simulink model "sgMdl_IO145_AnalogDigitalLoopback"  (R2024b)
settings: Solver=FixedStepAuto  StartTime=0.0  StopTime=inf  RelTol=1e-3  EnableMultiTasking=on
libraries: speedgoatlib_IO145 x5
Description:
  | IO145 - Analog and Digital Loopback
settings Model: ModifiedByFormat=Speedgoat  SimulationMode=external  ExtModeEnableFloating=off  ExtModeTrigDuration=100000  Creator=Speedgoat  LastModifiedBy=Speedgoat
settings SolverCC: ConcurrentTasks=on  AlgebraicLoopSolver=TrustRegion  PositivePriorityOrder=on
settings DataIOCC: SaveFormat=StructureWithTime  ReturnWorkspaceOutputs=off
settings OptimizationCC: BlockReduction=off  OptimizeBlockIOStorage=off  BufferReuse=off  ReuseModelBlockBuffer=off  GlobalBufferReuse=off  ExpressionFolding=off  LocalBlockOutputs=off
settings DebuggingCC: TasksWithSamePriorityMsg=none  UnconnectedInputMsg=warning  UnconnectedOutputMsg=warning  UnconnectedLineMsg=warning  SFExecutionAtInitializationDiag=none  ArithmeticOperatorsInVariantConditions=warning
settings HardwareCC: ProdBitPerLong=64  ProdLongLongMode=on  ProdHWDeviceType=Intel->x86-64 (Linux 64)
settings ModelReferenceCC: EnableRefExpFcnMdlSchedulingChecks=on
settings SFSimCC: SimUseLocalCustomCode=off  CustomCodeUndefinedFunction=UseInterfaceOnly
settings RTWCC: Description=Speedgoat Real-Time Target Machine  SystemTargetFile=speedgoat.tlc  TemplateMakefile=slrealtime_default_tmf  RTWUseLocalCustomCode=off  Toolchain=Simulink Real-Time Toolchain  BuildConfiguration=Faster Runs  TargetLang=C++  GPUComputeCapability=3.5  DLArmComputeVersion=19.05
settings CodeAppCC: StateflowObjectComments=on
settings SimulinkRealTimeTargetCC: SubcomponentCodeInterfacePackaging=Reusable function  InstructionSetFMA=off  LogToMDFFile=off  SLRTFileLogMaxRuns=10  UseGCCFastMath=on
settings ConfigComp: CovBoundaryAbsTol=1.0e-5
settings SimscapeCC: SimscapeNormalizeSystem=off

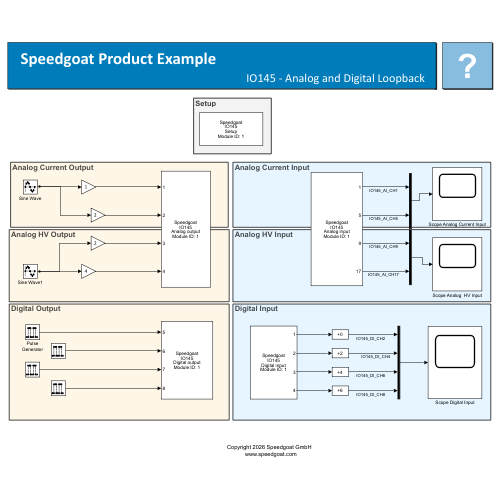
[thumbnail: Simulink's stored preview of the top-level diagram]
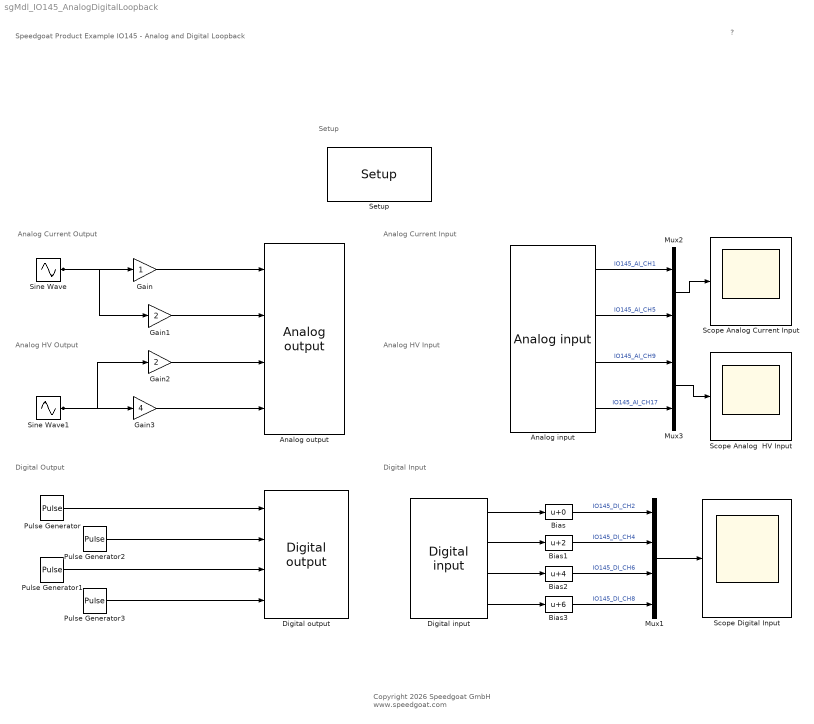
== system sgMdl_IO145_AnalogDigitalLoopback ==
  note: Digital Input
  note: Analog HV Input
  note: Analog HV Output
  note: Digital Output
  note: Setup
  note: Analog Current Output
  note: Analog Current Input
  note: Speedgoat Product Example
      | IO145 - Analog and Digital Loopback
  note: ?
  note: Copyright 2026 Speedgoat GmbH
      |  www.speedgoat.com
  "Analog input " : speedgoatlib_IO145/Analog input   parModuleId=1  parSampleTime=-1  parPciSlot=-1  parAdcChannels=[1 9 17 25]  parAdcNumActiveChannels=[1 1 1 1]  parAdcVoltageRange=[1 1 1 1 1 1 1 1 1 1 1 1 1 1 1 1 1 1 1 1 1 1 1 1 1 1 1 1 1 1 1 1]  parAdcCoupling=[1 1 1 1]  parAdcContSampling=0  parAdcDmaEnable=0  parAdcActiveDmaDevices=[1 1 1 1]  parAdcFrameSize=100
      settings: SourceProductName=Simulink Real-Time: Speedgoat I/O Blockset
  "Analog output " : speedgoatlib_IO145/Analog output   parModuleId=1  parSampleTime=-1  parPciSlot=-1  parDacChannels=[1 2 3 4]  parDacVoltageRange=[10 10 7 7 7 7 1 1]  parDacOverRange=[0 0 0 0 0 0 0 0]  parDacInitValues=[0 0 0 0]  parDacReset=[1 1 1 1]  parDacSyncOut=1  parDacDmaEnable=0  parDacActiveDmaDevices=[1 1 1 1]  parDacDmaLatency=2  parDacFrameSize=100
      settings: SourceProductName=Simulink Real-Time: Speedgoat I/O Blockset
  Bias : Bias  SaturateOnIntegerOverflow=off
  Bias1 : Bias  Bias=2  SaturateOnIntegerOverflow=off
  Bias2 : Bias  Bias=4  SaturateOnIntegerOverflow=off
  Bias3 : Bias  Bias=6  SaturateOnIntegerOverflow=off
  "Digital input " : speedgoatlib_IO145/Digital input   parModuleId=1  parSampleTime=-1  parPciSlot=-1  parDiChannels=[2 4 6 8]
      settings: SourceProductName=Simulink Real-Time: Speedgoat I/O Blockset
  "Digital output " : speedgoatlib_IO145/Digital output   parModuleId=1  parSampleTime=-1  parPciSlot=-1  parDoChannels=[1 3 5 7]  parDoInitValues=[0 0 0 0]  parDoReset=[1 1 1 1]
      settings: SourceProductName=Simulink Real-Time: Speedgoat I/O Blockset
  Gain : Gain
  Gain1 : Gain  Gain=2
  Gain2 : Gain  Gain=2
  Gain3 : Gain  Gain=4
  Mux1 : Mux
  Mux2 : Mux  Inputs=2
  Mux3 : Mux  Inputs=2
  Pulse Generator : DiscretePulseGenerator  Period=25  PulseWidth=5  SampleTime=0.001
  Pulse Generator1 : DiscretePulseGenerator  Period=25  PulseWidth=15  SampleTime=0.001
  Pulse Generator2 : DiscretePulseGenerator  Period=25  PulseWidth=10  SampleTime=0.001
  Pulse Generator3 : DiscretePulseGenerator  Period=25  PulseWidth=20  SampleTime=0.001
  Scope Analog  HV Input : Scope
  Scope Analog Current Input : Scope
  Scope Digital Input : Scope
  "Setup " : speedgoatlib_IO145/Setup   parPciSlot=-1  parModuleId=1  parInterModuleSync=Independent  parConvClockBaseRate=20MHz  parConvClock1Divider=20000  parConvClock2Divider=20000  parFrameTriggerEnable=off  parFrameTriggerDivider=10  parConvClock1BaseRate=1  parConvClock2BaseRate=1  parFrameTriggerClock=1  parAdcCoupling1=Differential  parAdcChannels1=[1 2]  parAdcChannel11=on  parAdcChannel12=off  parAdcChannel13=off  parAdcChannel14=off  parAdcChannel15=off  parAdcChannel16=off  parAdcChannel17=off  parAdcChannel18=off  parAdcRangeAll1=+-25 mA  parVoltageRangePerChannelEn1=off  parAdcRange11=+-25 mA  parAdcRange12=+-25 mA  parAdcRange13=+-25 mA  parAdcRange14=+-25 mA  parAdcRange15=+-25 mA  parAdcRange16=+-25 mA  parAdcRange17=+-25 mA  parAdcRange18=+-25 mA  parAdcCoupling2=Differential  parAdcChannels2=[9 10]  parAdcChannel21=on  parAdcChannel22=off  parAdcChannel23=off  parAdcChannel24=off  parAdcChannel25=off  parAdcChannel26=off  parAdcChannel27=off  parAdcChannel28=off  parAdcRangeAll2=+-25 mA  parVoltageRangePerChannelEn2=off  parAdcRange21=+-25 mA  parAdcRange22=+-25 mA  parAdcRange23=+-25 mA  parAdcRange24=+-25 mA  parAdcRange25=+-25 mA  parAdcRange26=+-25 mA  parAdcRange27=+-25 mA  parAdcRange28=+-25 mA  parAdcCoupling3=Differential  parAdcChannels3=[17 18]  parAdcChannel31=on  parAdcChannel32=off  parAdcChannel33=off  parAdcChannel34=off  parAdcChannel35=off  parAdcChannel36=off  parAdcChannel37=off  parAdcChannel38=off  parAdcRangeAll3=+-10V  parVoltageRangePerChannelEn3=off  parAdcRange31=+-20V  parAdcRange32=+-10V  parAdcRange33=+-10V  parAdcRange34=+-10V  parAdcRange35=+-10V  parAdcRange36=+-10V  parAdcRange37=+-10V  parAdcRange38=+-10V  parAdcCoupling4=Differential  parAdcChannels4=[25 26]  parAdcChannel41=on  parAdcChannel42=off  parAdcChannel43=off  parAdcChannel44=off  parAdcChannel45=off  parAdcChannel46=off  parAdcChannel47=off  parAdcChannel48=off  parAdcRangeAll4=+-10V  parVoltageRangePerChannelEn4=off  parAdcRange41=+-10V  parAdcRange42=+-10V  parAdcRange43=+-10V  parAdcRange44=+-10V  parAdcRange45=+-10V  parAdcRange46=+-10V  parAdcRange47=+-10V  parAdcRange48=+-10V  parAdcChannels=[1 9 17 25]  parAdcNumActiveChannels=[1 1 1 1]  parAdcVoltageRange=[1 1 1 1 1 1 1 1 1 1 1 1 1 1 1 1 1 1 1 1 1 1 1 1 1 1 1 1 1 1 1 1]  parAdcCoupling=[1 1 1 1]  parAdcContSampling=off  parAdcAutoCorrection=on  parAdcDmaEnable=off  parAdcDmaClock=Clock 1  parAdcFrameSize_=100  parAdcSampleTime_=-1  parAdcActiveDmaDevices=[1 1 1 1]  parAdcFrameTriggerEnable=0  parAdcFrameSize=100  parAdcSampleTime=0.1  parDacChannels=[1 2 3 4]  parDacChannel1=on  parDacChannel2=on  parDacChannel3=on  parDacChannel4=on  parDacChannel5=off  parDacChannel6=off  parDacChannel7=off  parDacChannel8=off  parDacInitValues=0  parDacResets=1  parDacVoltageRange=[10 10 7 7 7 7 1 1]  parDacOverRange=[0 0 0 0 0 0 0 0]  parDacRange1=0-20 mA  parDacInitValue1=0  parDacReset1=on  parDacRange2=0-20 mA  parDacInitValue2=0  parDacReset2=on  parDacRange3=+-10 V  parDacInitValue3=0  parDacReset3=on  parDacRange4=+-10 V  parDacInitValue4=0  parDacReset4=on  parDacRange5=+-10 V  parDacInitValue5=0  parDacReset5=on  parDacRange6=+-10 V  parDacInitValue6=0  parDacReset6=on  parDacRange7=0-5 V  parDacInitValue7=0  parDacReset7=on  parDacRange8=0-5 V  parDacInitValue8=0  parDacReset8=on  parDacAutoCorrection=on  parDacSyncOut=on  parDacDmaEnable=off  parDacDmaLatency=Until next frame  parDacDmaClock=Clock 1  parDacFrameSize_=100  parDacSampleTime_=-1  parDacActiveDmaDevices=[1 1 1 1]  parDacFrameTriggerEnable=0  parDacFrameSize=100  parDacSampleTime=0.1  parDiChannels=[2 4 6 8]  parDoChannels=[1 3 5 7]  parDioChannel1=Out  parDioChannel2=In  parDioChannel3=Out  parDioChannel4=In  parDioChannel5=Out  parDioChannel6=In  parDioChannel7=Out  parDioChannel8=In  parDoInitValues=[0 0 0 0]  parDoReset=[1 1 1 1]  parDoInitValue1=0  parDoReset1=on  parDoInitValue2=0  parDoReset2=on  parDoInitValue3=0  parDoReset3=on  parDoInitValue4=0  parDoReset4=on  parDoInitValue5=0  parDoReset5=on  parDoInitValue6=0  parDoReset6=on  parDoInitValue7=0  parDoReset7=on  parDoInitValue8=0  parDoReset8=on  parDiDebounceEnable=off  parDiDebounceTime=0  parDiDebounceValue=0  parDioPullRefFront=Floating  parDioPullRefRear=Floating
      settings: SourceProductName=Simulink Real-Time: Speedgoat I/O Blockset
  Sine Wave : Sin  SineType=Sample based  Amplitude=0.0005  Frequency=2*pi*5  Samples=50  SampleTime=0.001
  Sine Wave1 : Sin  SineType=Sample based  Frequency=2*pi*5  Samples=50  SampleTime=0.001
  wires:
  Gain/1 -> "Analog output "/1
  Gain3/1 -> "Analog output "/4
  Sine Wave/1 -> Gain1/1, Gain/1
  "Analog input "/2 -> Mux2/2  "IO145_AI_CH5"
  "Analog input "/1 -> Mux2/1  "IO145_AI_CH1"
  "Analog input "/4 -> Mux3/2  "IO145_AI_CH17"
  "Analog input "/3 -> Mux3/1  "IO145_AI_CH9"
  Gain2/1 -> "Analog output "/3
  Gain1/1 -> "Analog output "/2
  Pulse Generator3/1 -> "Digital output "/4
  Pulse Generator1/1 -> "Digital output "/3
  Pulse Generator2/1 -> "Digital output "/2
  Pulse Generator/1 -> "Digital output "/1
  Mux1/1 -> Scope Digital Input/1
  Bias/1 -> Mux1/1  "IO145_DI_CH2"
  Bias1/1 -> Mux1/2  "IO145_DI_CH4"
  Bias2/1 -> Mux1/3  "IO145_DI_CH6"
  Bias3/1 -> Mux1/4  "IO145_DI_CH8"
  Mux2/1 -> Scope Analog Current Input/1
  "Digital input "/1 -> Bias/1
  "Digital input "/2 -> Bias1/1
  "Digital input "/3 -> Bias2/1
  "Digital input "/4 -> Bias3/1
  Sine Wave1/1 -> Gain2/1, Gain3/1
  Mux3/1 -> Scope Analog  HV Input/1
